simulink model "Delay_Counter"  (R2024b)
settings: Solver=FixedStepAuto  StartTime=0.0  StopTime=10  FixedStep=0.5  RelTol=1e-3
settings Model: Creator=abdal  LastModifiedBy=abdal

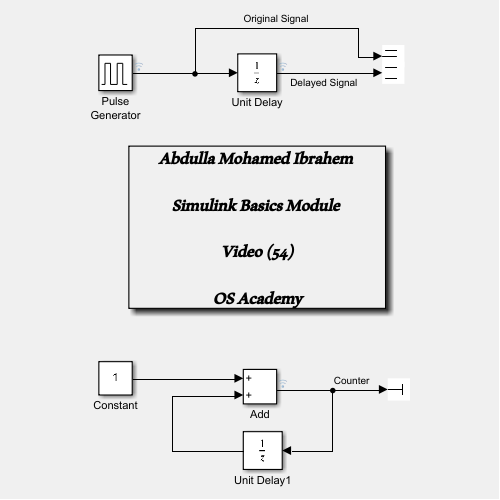
[thumbnail: Simulink's stored preview of the top-level diagram]
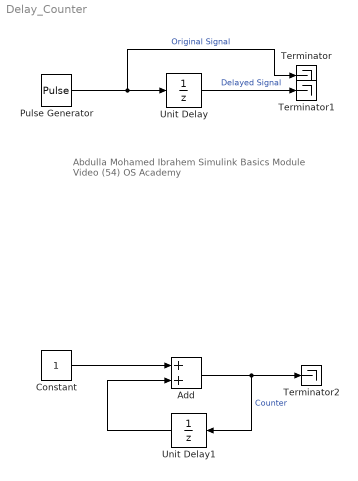
== system Delay_Counter ==
  note: Abdulla Mohamed Ibrahem
      | Simulink Basics Module
      | Video (54)
      | OS Academy
  Add : Sum
  Constant : Constant
  Pulse Generator : DiscretePulseGenerator  PulseType=Time based  Period=1  PulseWidth=50
  Terminator : Terminator
  Terminator1 : Terminator
  Terminator2 : Terminator
  Unit Delay : UnitDelay  SampleTime=-1  HasFrameUpgradeWarning=on
  Unit Delay1 : UnitDelay  SampleTime=-1  HasFrameUpgradeWarning=on
  wires:
  Unit Delay/1 -> Terminator1/1  "Delayed Signal"
  Pulse Generator/1 -> Terminator/1, Unit Delay/1  "Original Signal"
  Constant/1 -> Add/1
  Add/1 -> Terminator2/1, Unit Delay1/1  "Counter"
  Unit Delay1/1 -> Add/2
